simulink model "gtcs_model_and_controller"  (R2021a)
settings: Solver=VariableStepAuto  StartTime=0.0  StopTime=10  RelTol=1e-3
InitFcn:
  | load('param_motor.mat');
  | load('param_controller_2.mat');
values from neighbouring files (symbols this model uses):
  K_t = 0.0375    [param_motor.mat]
libraries: fl_lib x21, nesl_utility x13, ee_lib x10, sdl_lib x4
settings Model: Creator=ANKARA-OFIS  LastModifiedBy=ANKARA-OFIS

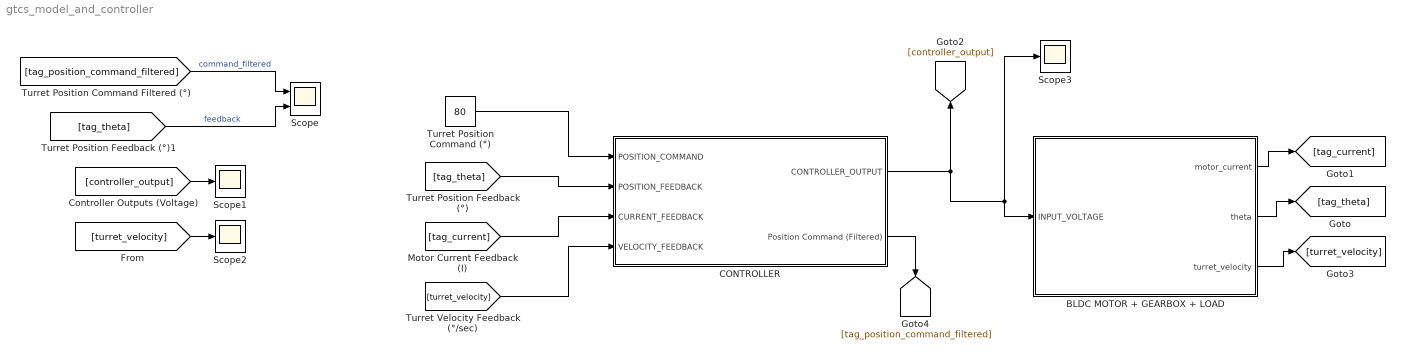
== system gtcs_model_and_controller ==
  BLDC MOTOR + GEARBOX + LOAD : Subsystem
  CONTROLLER : Subsystem
  Scope : Scope  NumInputPorts=2
  Scope1 : Scope
  Scope2 : Scope
  Scope3 : Scope
  Turret Position Command (°) : Constant  Value=80
  wires:
  Turret Position Command (°)/1 -> CONTROLLER/1(POSITION_COMMAND)
  [tag_theta] -> CONTROLLER/2(POSITION_FEEDBACK)
  [tag_current] -> CONTROLLER/3(CURRENT_FEEDBACK)
  BLDC MOTOR + GEARBOX + LOAD/2(theta) -> [tag_theta]
  BLDC MOTOR + GEARBOX + LOAD/1(motor_current) -> [tag_current]
  BLDC MOTOR + GEARBOX + LOAD/3(turret_velocity) -> [turret_velocity]
  [turret_velocity] -> CONTROLLER/4(VELOCITY_FEEDBACK)
  [turret_velocity] -> Scope2/1
  [controller_output] -> Scope1/1
  [tag_theta] -> Scope/2  "feedback"
  [tag_position_command_filtered] -> Scope/1  "command_filtered"
  CONTROLLER/2(Position Command (Filtered)) -> [tag_position_command_filtered]
  CONTROLLER/1(CONTROLLER_OUTPUT) -> Scope3/1, BLDC MOTOR + GEARBOX + LOAD/1(INPUT_VOLTAGE), [controller_output]

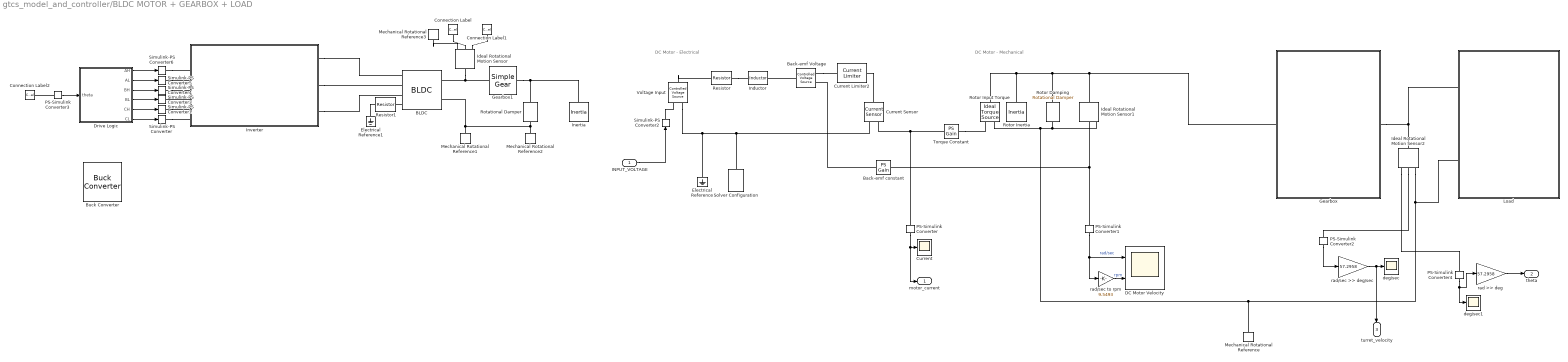
== system gtcs_model_and_controller/BLDC MOTOR + GEARBOX + LOAD ==
  note: DC Motor - Mechanical
  note: DC Motor - Electrical
  INPUT_VOLTAGE : Inport
  BLDC : ee_lib/Electromechanical/Permanent Magnet/BLDC  winding_type=ee.enum.statorconnection.wye  rotor_param=ee.enum.pmsm.backemf.trapezoidflux  pm_flux_linkage=0.03 Wb  theta_constant=pi / 12 rad  emf_max=9.6 V  DphiDtheta_tab=[0, -.1528, -.1528, .1528, .1528, 0] Wb/rad  back_emf_tab=[0, -9.6, -9.6, 9.6, 9.6, 0] V  rotor_angle_tab=[0, 7.5, 22.5, 37.5, 52.5, 60] deg  w_meas=600 rpm  nPolePairs=6  stator_param=ee.enum.statorparam.LdLqL0  machine_param=ee.enum.dqparameterization.constant  Ld=0.00022 H  Lq=0.00022 H  idVec=[-200, 0, 200] A  iqVec=[-200, 0, 200] A  LdMatrix=0.00022 * ones(3, 3) H  LqMatrix=0.00022 * ones(3, 3) H  L0=0.00016 H  Ls=0.0002 H  Lm=0 H  Ms=0.00002 H  Rs=0.013 Ohm  zero_sequence=ee.enum.park.zerosequence.include  J=0.01 kg*m^2  lam=0 N*m/(rad/s)  axes_param=ee.enum.rotorangle.daxis  i_d_specify=off  i_d_priority=None  i_d=0 A  i_d_nominal_specify=off  i_d_nominal_unit=A  i_d_nominal_value=1  i_q_specify=off  i_q_priority=None  i_q=0 A  i_q_nominal_specify=off  i_q_nominal_unit=A  i_q_nominal_value=1  torque_specify=off  torque_priority=None  torque=0 N*m  torque_nominal_specify=off  torque_nominal_unit=N*m  torque_nominal_value=1  angular_velocity_specify=off  angular_velocity_priority=High  angular_velocity=0 rpm  angular_velocity_nominal_specify=off  angular_velocity_nominal_unit=rpm  angular_velocity_nominal_value=1  angular_position_specify=off  angular_position_priority=High  angular_position=0 deg  angular_position_nominal_specify=off  angular_position_nominal_unit=deg  angular_position_nominal_value=1  loss_param=ee.enum.ironloss.none  losses_oc=[0, 0, 0] W  losses_sc=[0, 0, 0] W  f_losses=60 Hz  Isc_losses=95 A  Tmeas=298.15 K  alpha=3.93e-3 1/K  alpha_flux=-0.001 1/K  stator_thermal_mass=100 J/K  rotor_thermal_mass=200 J/K  Rm_percent_rotor=90  Rd_percent_rotor=30  temperatureA_specify=off  temperatureA_priority=High  temperatureA=25 degC  temperatureA_nominal_specify=off  temperatureA_nominal_unit=degC  temperatureA_nominal_value=1  temperatureB_specify=off  temperatureB_priority=High  temperatureB=25 degC  temperatureB_nominal_specify=off  temperatureB_nominal_unit=degC  temperatureB_nominal_value=1  temperatureC_specify=off  temperatureC_priority=High  temperatureC=25 degC  temperatureC_nominal_specify=off  temperatureC_nominal_unit=degC  temperatureC_nominal_value=1  temperatureR_specify=off  temperatureR_priority=High  temperatureR=25 degC  temperatureR_nominal_specify=off  temperatureR_nominal_unit=degC  temperatureR_nominal_value=1
      settings: SourceProductBaseCode=PS  InternalSimscapePortConfiguration="{\"Bottom\":[],\"Left\":[{\"id\":\"a\",\"label\":\"a\",\"type\":\"foundation.electrical.electrical\"},{\"id\":\"b\",\"label\":\"b\",\"type\":\"foundation.electrical.electrical\"},{\"id\":\"c\",\"label\":\"c\",\"type\":\"foundation.electrical.electrical\"},{\"id\":\"n\",\"label\":\"n\",\"type\":\"foundation.electrical.electrical\"}],\"Right\":[{\"id\":\"R\",\"label\":\"R\",\"type\":\"foundation.mechanical.rotational.rotational\"},{\"id\":\"C\",\"label\":\"C\",\"type\":\"foundation.mechanical.rotational.rotational\"}],\"Top\":[]}"
  Back-emf Voltage : fl_lib/Electrical/Electrical Sources/Controlled Voltage Source
  Back-emf constant : fl_lib/Physical Signals/Functions/PS Gain  gain=0.04 V*s/rad
  Buck Converter : ee_lib/Semiconductors & Converters/Converters/Buck Converter  device_type=ee.enum.converters.switchingdevice.ideal  Vf=0.8 V  Ron=0.001 Ohm  Rds=0.001 Ohm  Goff=1e-5 1/Ohm  Vth=6 V  Vgt=1 V  Vgt_off=-1 V  Ih=1 A  diode_param=ee.enum.converters.protectiondiode.nodynamics  diode_Vf=0.8 V  diode_Ron=0.001 Ohm  diode_Goff=1e-5 1/Ohm  diode_C=50 nF  diode_iRM=-235 A  diode_iF=300 A  diode_idot=-50 A/us  diode_trr_param=ee.enum.converters.diodetrr.trr_factor  diode_trr_factor=3  diode_trr=15 us  diode_Qrr=1500 s*uA  Lf=1e-6 H  Rl=0 Ohm  Cf=1e-7 F  Rf=1e-6 Ohm  snubber_type=ee.enum.converters.snubber.exclude  Rs=0.1 Ohm  Cs=1e-7 F  iL_specify=off  iL_priority=High  iL=0 A  iL_nominal_specify=off  iL_nominal_unit=A  iL_nominal_value=1  vc_specify=off  vc_priority=High  vc=0 V  vc_nominal_specify=off  vc_nominal_unit=V  vc_nominal_value=1
      settings: SourceProductBaseCode=PS  InternalSimscapePortConfiguration="{\"Bottom\":[],\"Left\":[{\"id\":\"G\",\"label\":\"G\",\"type\":\"input\"},{\"id\":\"p1\",\"label\":\"1+\",\"type\":\"foundation.electrical.electrical\"},{\"id\":\"n1\",\"label\":\"1-\",\"type\":\"foundation.electrical.electrical\"}],\"Right\":[{\"id\":\"p2\",\"label\":\"2+\",\"type\":\"foundation.electrical.electrical\"},{\"id\":\"n2\",\"label\":\"2-\",\"type\":\"foundation.electrical.electrical\"}],\"Top\":[]}"
  Connection Label : ConnectionLabel  Label=motor_omega
  Connection Label1 : ConnectionLabel  Label=motor_theta
  Connection Label2 : ConnectionLabel  Label=motor_theta
  Current : Scope
  Current Limiter2 : ee_lib/Semiconductors & Converters/Current Limiter  iLim=80 A  vLim=0.1 V  gLim=1e-3 1/Ohm  thermal_mass=100 J/K  initial_temperature=298.15 K
      settings: SourceProductBaseCode=PS  InternalSimscapePortConfiguration="{\"Bottom\":[],\"Left\":[{\"id\":\"p\",\"label\":\"+\",\"type\":\"foundation.electrical.electrical\"}],\"Right\":[{\"id\":\"n\",\"label\":\"-\",\"type\":\"foundation.electrical.electrical\"}],\"Top\":[]}"
  Current Sensor : fl_lib/Electrical/Electrical Sensors/Current Sensor
  DC Motor Velocity : Scope  NumInputPorts=2
  Drive Logic : MATLAB Function  TreatAsAtomicUnit=on
  Electrical Reference : fl_lib/Electrical/Electrical Elements/Electrical Reference
  Electrical Reference1 : fl_lib/Electrical/Electrical Elements/Electrical Reference
  Gearbox : Subsystem
  Gearbox1 : sdl_lib/Gears/Simple Gear  ratio=435.6  rotation_direction=sdl.enum.shaftOutputDirection.same  friction_model=sdl.enum.gear_efficiencies_load.off  mu_visc=[0, 0] N*m/(rad/s)  T_noload=0.1 N*m  T_nom=5 N*m  efficiency_nom=0.8  efficiency=0.8  temperature_TLU=[280, 300, 320] K  load_TLU=[1, 5, 10] N*m  efficiency_TLU=[.95, .9, .85]  efficiency_TLU2=[.85, .8, .75; .95, .9, .85; .85, .8, .7]  w_thr=0.01 rad/s  pwr_thr=0.001 W  thermal_mass=50 J/K  enable_faults=simscape.enum.onoff.off  efficiency_fault=0.05  external_fault=simscape.enum.onoff.off  temporal_fault=simscape.enum.onoff.off  fault_time=5 s  fault_angles=pi / 12 rad  report_fault=simscape.enum.assert.action.none  temperature_specify=off  temperature_priority=High  temperature=300 K  temperature_nominal_specify=off  temperature_nominal_unit=K  temperature_nominal_value=1
  Ideal Rotational Motion Sensor : fl_lib/Mechanical/Mechanical Sensors/Ideal Rotational Motion Sensor  wrap_angle=simscape.enum.onoff.off  offset=0 rad
  Ideal Rotational Motion Sensor1 : fl_lib/Mechanical/Mechanical Sensors/Ideal Rotational Motion Sensor  wrap_angle=simscape.enum.onoff.on  offset=0 rad
  Ideal Rotational Motion Sensor2 : fl_lib/Mechanical/Mechanical Sensors/Ideal Rotational Motion Sensor  wrap_angle=simscape.enum.onoff.off  offset=0 rad
  Inductor : ee_lib/Passive/Inductor  l=18e-6 H  L_tol=20  enable_L_tol=0  tol_distribution=1  nSigma=4  r=0 Ohm  g=1e-9 1/Ohm  enable_operating_limits=0  operating_limit_action=2  max_working_current=1 A  power_rating=1 W  enable_faults=0  fault_action=1  lambdaPercent=50  k_faulted=0.9999  turnsShort=0  openCct=0  groundShort=0  groundShortG=0 1/Ohm  tau_fault=1e-3 s  enable_temporal_fault=0  t_fault=1 s  enable_behavioral_fault=0  max_permissible_voltage=100 V  n_fail_on_voltage=1  max_permissible_current=1 A  t_fail_on_current=1 s  i_L_specify=off  i_L_priority=High  i_L=0 A  i_L_nominal_specify=off  i_L_nominal_unit=A  i_L_nominal_value=1
  Inertia : fl_lib/Mechanical/Rotational Elements/Inertia  inertia=0.01 kg*m^2  num_ports=foundation.enum.numPorts2.one  w_specify=off  w_priority=High  w=0 rad/s  w_nominal_specify=off  w_nominal_unit=rad/s  w_nominal_value=1  t_specify=off  t_priority=None  t=0 N*m  t_nominal_specify=off  t_nominal_unit=N*m  t_nominal_value=1
  Inverter : Subsystem
  Load : Subsystem
  Mechanical Rotational Reference{,1..3} (4 alike) : fl_lib/Mechanical/Rotational Elements/Mechanical Rotational Reference
  PS-Simulink Converter{,1..4} (5 alike) : nesl_utility/PS-Simulink Converter  PhysicalDomain=network_engine_domain  SubClassName=ps_output  LeftPortType=input  RightPortType=output  PseudoPeriodic=off  Frequencies=[]  Unit=inherit  AffineConversion=off
      settings: SourceProductBaseCode=PW,SS
  Resistor : fl_lib/Electrical/Electrical Elements/Resistor  R=45e-03 Ohm  i_specify=off  i_priority=None  i=0 A  i_nominal_specify=off  i_nominal_unit=A  i_nominal_value=1  v_specify=off  v_priority=None  v=0 V  v_nominal_specify=off  v_nominal_unit=V  v_nominal_value=1
  Resistor1 : fl_lib/Electrical/Electrical Elements/Resistor  R=1 Ohm  i_specify=off  i_priority=None  i=0 A  i_nominal_specify=off  i_nominal_unit=A  i_nominal_value=1  v_specify=off  v_priority=None  v=0 V  v_nominal_specify=off  v_nominal_unit=V  v_nominal_value=1
  Rotational Damper : sdl_lib/Couplings & Drives/Springs & Dampers/Rotational Damper  D=1e-3 N*m/(rad/s)  enable_faults=0  b_fault=100 N*m/(rad/s)  temporal_fault=0  fault_time=5 s  shock_fault=0  acceleration_limit=100 rad/s^2  shock_limit=1  report_fault=1
      settings: SourceProductBaseCode=LD
  Rotor Damping : fl_lib/Mechanical/Rotational Elements/Rotational Damper  D=0.0001 N*m/(rad/s)  w_specify=off  w_priority=None  w=0 rad/s  w_nominal_specify=off  w_nominal_unit=rad/s  w_nominal_value=1  t_specify=off  t_priority=None  t=0 N*m  t_nominal_specify=off  t_nominal_unit=N*m  t_nominal_value=1
  Rotor Inertia : fl_lib/Mechanical/Rotational Elements/Inertia  inertia=100 kg*mm^2  num_ports=foundation.enum.numPorts2.one  w_specify=off  w_priority=High  w=0 rad/s  w_nominal_specify=off  w_nominal_unit=rad/s  w_nominal_value=1  t_specify=off  t_priority=None  t=0 N*m  t_nominal_specify=off  t_nominal_unit=N*m  t_nominal_value=1
  Rotor Input Torque : fl_lib/Mechanical/Mechanical Sources/Ideal Torque Source
  Simulink-PS Converter{,1..6} (7 alike) : nesl_utility/Simulink-PS Converter  PhysicalDomain=network_engine_domain  SubClassName=ps_input  LeftPortType=input  RightPortType=output  PseudoPeriodic=off  Frequencies=[]  NoiseDistribution=none  NoiseParameters=[]  Unit=1  AffineConversion=off  FilteringAndDerivatives=provide  SimscapeFilterOrder=1  InputFilterTimeConstant=0.001  UdotUserProvided=0
      settings: SourceProductBaseCode=PW,SS
  Solver Configuration : nesl_utility/Solver Configuration  PhysicalDomain=network_engine_domain  SubClassName=solver  LeftPortType=input  RightPortType=generic  Tones=[]  Harmonics=[]  SimulateNoise=off  Profile=off  UseLocalSampling=off  EnableSwitchedLinearOptims=on  FrequencyDomain=off  UseCCode=off  RelTol=0.001  AbsTol=1e-06  MinStep=1e-09  ToWorkspace=off  RevertToSquareIcSolve=off  NumHomotopyIterations=100  PhasorMode=off  PhasorModeNumHarmonics=1  DoDC=off  ResidualTolerance=1e-09  UseLocalSolver=off  LocalSolverChoice=NE_BACKWARD_EULER_ADVANCER  LocalSolverSampleTime=0.001  DoFixedCost=off  MaxNonlinIter=3  MaxModeIter=2  ComputeImpulses=off  ImpulseIterations=2  LinearAlgebra=auto  EquationFormulation=NE_TIME_EF  DelaysMemoryBudget=1024  AutomaticFiltering=on  FilteringTimeConstant=0.001  PartitionStorageMethod=AS_NEEDED  PartitionMemoryBudget=1024  PartitionMethod=ROBUST
      settings: SourceProductBaseCode=PW,SS
  Torque Constant : fl_lib/Physical Signals/Functions/PS Gain  gain=K_t N*m/A
  Voltage Input : fl_lib/Electrical/Electrical Sources/Controlled Voltage Source
  deg/sec : Scope
  deg/sec1 : Scope
  rad >> deg : Gain  Gain=57.2958
  rad/sec >> deg/sec : Gain  Gain=57.2958
  rad/sec to rpm : Gain  Gain=9.5493
  motor_current : Outport
  theta : Outport  Port=2
  turret_velocity : Outport  Port=3
  wires:
  PS-Simulink Converter2/1 -> rad/sec >> deg/sec/1
  INPUT_VOLTAGE/1 -> Simulink-PS Converter2/1
  PS-Simulink Converter/1 -> motor_current/1, Current/1
  PS-Simulink Converter1/1 -> DC Motor Velocity/1, rad/sec to rpm/1  "rad/sec"
  rad/sec to rpm/1 -> DC Motor Velocity/2  "rpm"
  rad/sec >> deg/sec/1 -> turret_velocity/1, deg/sec/1
  PS-Simulink Converter4/1 -> rad >> deg/1, deg/sec1/1
  rad >> deg/1 -> theta/1
  PS-Simulink Converter3/1 -> Drive Logic/1(theta)
  Drive Logic/6(CL) -> Simulink-PS Converter/1
  Drive Logic/5(CH) -> Simulink-PS Converter1/1
  Drive Logic/4(BL) -> Simulink-PS Converter3/1
  Drive Logic/3(BH) -> Simulink-PS Converter4/1
  Drive Logic/2(AL) -> Simulink-PS Converter5/1
  Drive Logic/1(AH) -> Simulink-PS Converter6/1
  connections:
  Rotor Damping/LConn1 -- Rotor Input Torque/LConn1 -- Rotor Inertia/LConn1 -- Gearbox/LConn1 -- Ideal Rotational Motion Sensor1/LConn1
  Mechanical Rotational Reference/LConn1 -- Rotor Damping/RConn1 -- Ideal Rotational Motion Sensor1/RConn1 -- Rotor Input Torque/RConn2 -- Ideal Rotational Motion Sensor2/RConn1 -- Load/LConn2
  Ideal Rotational Motion Sensor2/RConn2 -- PS-Simulink Converter2/LConn1
  Torque Constant/RConn1 -- Rotor Input Torque/RConn1
  Ideal Rotational Motion Sensor1/RConn2 -- PS-Simulink Converter1/LConn1 -- Back-emf constant/LConn1
  Voltage Input/RConn1 -- Simulink-PS Converter2/RConn1
  Resistor/RConn1 -- Inductor/LConn1
  Current Limiter2/RConn1 -- Current Sensor/LConn1
  Voltage Input/LConn1 -- Resistor/LConn1
  Back-emf Voltage/RConn2 -- Current Limiter2/LConn1
  Torque Constant/LConn1 -- Current Sensor/RConn1 -- PS-Simulink Converter/LConn1
  Back-emf constant/RConn1 -- Back-emf Voltage/RConn1
  Back-emf Voltage/LConn1 -- Inductor/RConn1
  Electrical Reference/LConn1 -- Voltage Input/RConn2 -- Solver Configuration/RConn1 -- Current Sensor/RConn2
  Gearbox/RConn1 -- Load/LConn1 -- Ideal Rotational Motion Sensor2/LConn1
  Ideal Rotational Motion Sensor2/RConn3 -- PS-Simulink Converter4/LConn1
  Inverter/RConn2 -- BLDC/LConn2
  Inverter/RConn3 -- BLDC/LConn3
  Resistor1/LConn1 -- BLDC/LConn4
  Electrical Reference1/LConn1 -- Resistor1/RConn1
  Rotational Damper/LConn1 -- Gearbox1/RConn1 -- Inertia/LConn1
  Gearbox1/LConn1 -- Ideal Rotational Motion Sensor/LConn1 -- BLDC/RConn1
  Mechanical Rotational Reference1/LConn1 -- Rotational Damper/RConn1 -- Mechanical Rotational Reference2/LConn1 -- BLDC/RConn2
  Mechanical Rotational Reference3/LConn1 -- Ideal Rotational Motion Sensor/RConn1
  Connection Label/LConn1 -- Ideal Rotational Motion Sensor/RConn2
  Connection Label1/LConn1 -- Ideal Rotational Motion Sensor/RConn3
  Inverter/RConn1 -- BLDC/LConn1
  PS-Simulink Converter3/LConn1 -- Connection Label2/LConn1
  Simulink-PS Converter/RConn1 -- Inverter/LConn8
  Simulink-PS Converter1/RConn1 -- Inverter/LConn7
  Simulink-PS Converter3/RConn1 -- Inverter/LConn6
  Simulink-PS Converter4/RConn1 -- Inverter/LConn5
  Simulink-PS Converter5/RConn1 -- Inverter/LConn4
  Simulink-PS Converter6/RConn1 -- Inverter/LConn3

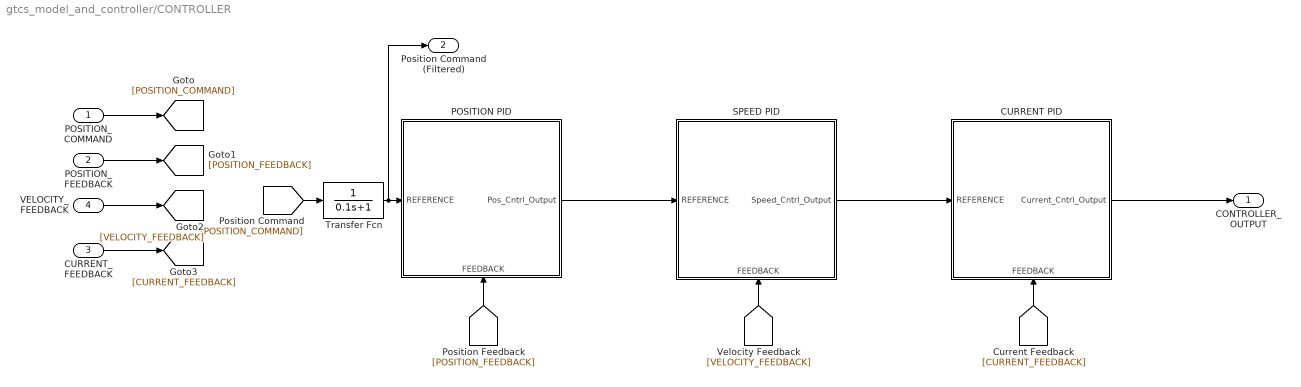
== system gtcs_model_and_controller/CONTROLLER ==
  POSITION_COMMAND : Inport
  POSITION_FEEDBACK : Inport  Port=2
  CURRENT_FEEDBACK : Inport  Port=3
  VELOCITY_FEEDBACK : Inport  Port=4
  CURRENT PID : Subsystem
      settings: PortSchema="{\"entries\":[{\"content\":{\"sides\":[{\"content\":{\"connectorIds\":[\"In1\"]},\"type\":\"ConnectorPlacement.EquallySpacedRectSide\",\"uuid\":\"40c65be9-b241-43d3-b74e-061528d6863f\"},{\"content\":{\"connectorIds\":[\"Out1\"],\"side\":\"RIGHT\"},\"type\":\"ConnectorPlacement.EquallySpacedRectSide\",\"uuid\":\"f0c37777-6186-40ca-93fa-111567e4da2a\"},{\"content\":{\"connectorIds\":[],\"side\":\"TOP\"},\"type\":\"ConnectorPlacement.EquallySpacedRectSide\",\"uuid\":\"f72b91dc-29bd-47db-bfb1-a15381258f12\"},{\"content\":{\"connectorIds\":[\"In2\"],\"side\":\"BOTTOM\"},\"type\":\"ConnectorPlacement.EquallySpacedRectSide\",\"uuid\":\"2008c998-139c-4ab5-8b80-fe5598144eb1\"}]},\"type\":\"ConnectorPlacement.EquallySpacedConnector\",\"uuid\":\"6c18c1ed-cfc3-452d-a661-af16ec8cef93\"}],\"packageUris\":[\"http://schema.mathworks.com/mf0/Connector/R2020b\"],\"version\":\"1.0\"}"
  POSITION PID : Subsystem
      settings: PortSchema="{\"entries\":[{\"content\":{\"sides\":[{\"content\":{\"connectorIds\":[\"In1\"]},\"type\":\"ConnectorPlacement.EquallySpacedRectSide\",\"uuid\":\"40c65be9-b241-43d3-b74e-061528d6863f\"},{\"content\":{\"connectorIds\":[\"Out1\"],\"side\":\"RIGHT\"},\"type\":\"ConnectorPlacement.EquallySpacedRectSide\",\"uuid\":\"f0c37777-6186-40ca-93fa-111567e4da2a\"},{\"content\":{\"connectorIds\":[],\"side\":\"TOP\"},\"type\":\"ConnectorPlacement.EquallySpacedRectSide\",\"uuid\":\"f72b91dc-29bd-47db-bfb1-a15381258f12\"},{\"content\":{\"connectorIds\":[\"In2\"],\"side\":\"BOTTOM\"},\"type\":\"ConnectorPlacement.EquallySpacedRectSide\",\"uuid\":\"2008c998-139c-4ab5-8b80-fe5598144eb1\"}]},\"type\":\"ConnectorPlacement.EquallySpacedConnector\",\"uuid\":\"6c18c1ed-cfc3-452d-a661-af16ec8cef93\"}],\"packageUris\":[\"http://schema.mathworks.com/mf0/Connector/R2020b\"],\"version\":\"1.0\"}"
  SPEED PID : Subsystem
      settings: PortSchema="{\"entries\":[{\"content\":{\"sides\":[{\"content\":{\"connectorIds\":[\"In1\"]},\"type\":\"ConnectorPlacement.EquallySpacedRectSide\",\"uuid\":\"40c65be9-b241-43d3-b74e-061528d6863f\"},{\"content\":{\"connectorIds\":[\"Out1\"],\"side\":\"RIGHT\"},\"type\":\"ConnectorPlacement.EquallySpacedRectSide\",\"uuid\":\"f0c37777-6186-40ca-93fa-111567e4da2a\"},{\"content\":{\"connectorIds\":[],\"side\":\"TOP\"},\"type\":\"ConnectorPlacement.EquallySpacedRectSide\",\"uuid\":\"f72b91dc-29bd-47db-bfb1-a15381258f12\"},{\"content\":{\"connectorIds\":[\"In2\"],\"side\":\"BOTTOM\"},\"type\":\"ConnectorPlacement.EquallySpacedRectSide\",\"uuid\":\"2008c998-139c-4ab5-8b80-fe5598144eb1\"}]},\"type\":\"ConnectorPlacement.EquallySpacedConnector\",\"uuid\":\"6c18c1ed-cfc3-452d-a661-af16ec8cef93\"}],\"packageUris\":[\"http://schema.mathworks.com/mf0/Connector/R2020b\"],\"version\":\"1.0\"}"
  Transfer Fcn : TransferFcn  Denominator=[0.1 1]
  CONTROLLER_OUTPUT : Outport
  Position Command (Filtered) : Outport  Port=2
  wires:
  POSITION_COMMAND/1 -> [POSITION_COMMAND]
  POSITION_FEEDBACK/1 -> [POSITION_FEEDBACK]
  VELOCITY_FEEDBACK/1 -> [VELOCITY_FEEDBACK]
  CURRENT_FEEDBACK/1 -> [CURRENT_FEEDBACK]
  [POSITION_COMMAND] -> Transfer Fcn/1
  [POSITION_FEEDBACK] -> POSITION PID/2(FEEDBACK)
  [VELOCITY_FEEDBACK] -> SPEED PID/2(FEEDBACK)
  [CURRENT_FEEDBACK] -> CURRENT PID/2(FEEDBACK)
  POSITION PID/1(Pos_Cntrl_Output) -> SPEED PID/1(REFERENCE)
  CURRENT PID/1(Current_Cntrl_Output) -> CONTROLLER_OUTPUT/1
  SPEED PID/1(Speed_Cntrl_Output) -> CURRENT PID/1(REFERENCE)
  Transfer Fcn/1 -> Position Command (Filtered)/1, POSITION PID/1(REFERENCE)

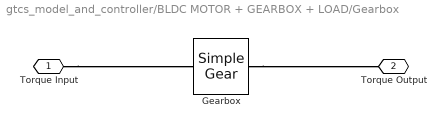
== system gtcs_model_and_controller/BLDC MOTOR + GEARBOX + LOAD/Gearbox ==
  Gearbox : sdl_lib/Gears/Simple Gear  ratio=435.6  rotation_direction=sdl.enum.shaftOutputDirection.same  friction_model=sdl.enum.gear_efficiencies_load.off  mu_visc=[0, 0] N*m/(rad/s)  T_noload=0.1 N*m  T_nom=5 N*m  efficiency_nom=0.8  efficiency=0.8  temperature_TLU=[280, 300, 320] K  load_TLU=[1, 5, 10] N*m  efficiency_TLU=[.95, .9, .85]  efficiency_TLU2=[.85, .8, .75; .95, .9, .85; .85, .8, .7]  w_thr=0.01 rad/s  pwr_thr=0.001 W  thermal_mass=50 J/K  enable_faults=simscape.enum.onoff.off  efficiency_fault=0.05  external_fault=simscape.enum.onoff.off  temporal_fault=simscape.enum.onoff.off  fault_time=5 s  fault_angles=pi / 12 rad  report_fault=simscape.enum.assert.action.none  temperature_specify=off  temperature_priority=High  temperature=300 K  temperature_nominal_specify=off  temperature_nominal_unit=K  temperature_nominal_value=1
  Torque Input : PMIOPort  Side=Left
  Torque Output : PMIOPort  Port=2  Side=Right
  connections:
  Gearbox/RConn1 -- Torque Output/RConn1
  Torque Input/RConn1 -- Gearbox/LConn1

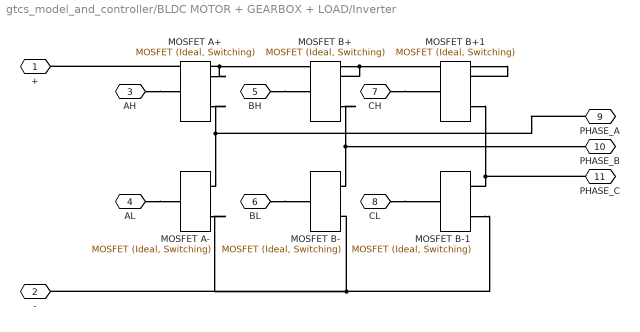
== system gtcs_model_and_controller/BLDC MOTOR + GEARBOX + LOAD/Inverter ==
  MOSFET A+ : ee_lib/Semiconductors & Converters/MOSFET (Ideal, Switching)  Rds=0.01 Ohm  Goff=1e-6 1/Ohm  Vth=2 V  diode_param=ee.enum.converters.protectiondiode.none  diode_Vf=0.8 V  diode_Ron=0.001 Ohm  diode_Goff=1e-5 1/Ohm  diode_C=50e-9 F  diode_iRM=-235 A  diode_iF=300 A  diode_idot=-50 A/us  diode_trr_param=ee.enum.converters.diodetrr.trr_factor  diode_trr_factor=3  diode_trr=15 us  diode_Qrr=1500 s*uA  thermal_loss_option=ee.enum.converters.thermalLossOption.constantvalues  Von_data=[0, 1.1, 1.3, 1.45, 1.75, 2.25, 2.7; 0, 1, 1.15, 1.35, 1.7, 2.35, 3] V  Eon_data=[0, .29, 1.43, 2.86, 5.71, 13.14, 22.86; 0, .57, 2.63, 5.14, 10.29, 20.57, 30.29] * 1e-3 J  Eoff_data=[0, .21, 1.07, 2.14, 4.29, 9.86, 17.14; 0, .43, 1.97, 3.86, 7.71, 15.43, 22.71] * 1e-3 J  Tj=[298.15, 398.15] K  Iout_data=[0, 10, 50, 100, 200, 400, 600] A  Eon_scalar=22.86e-3 J  Eoff_scalar=17.14e-3 J  Voff=300 V  Iout_scalar=600 A  diodeModelType=ee.enum.converters.diodeModelType.pwl  diode_IfMat=[.07, .12, .19, 1.75, 4.24, 7.32, 11.2; .16, .3, .72, 2.14, 4.02, 6.35, 9.12] A  diode_TjVec=[25, 125] degC  diode_VfVec=[.5, .7, .9, 1.3, 1.7, 2.1, 2.5] V  thermal_network_parameterization=ee.enum.thermalNetworkTopology.external  Rth=[.03, .2] K/W  Rth_Foster=[.03, .2] K/W  thermal_mass_parameterization=ee.enum.thermalNetwork.timeconstant  thermal_mass=[3, 25] J/K  thermal_mass_Foster=[33, 50] J/K  thermal_time_constant=[.1, 5] s  thermal_time_constant_Foster=[1, 10] s  thermal_mass_initial_temperatures=[25, 25] degC  junction_thermal_mass=0.1 J/K  vT_specify=off  vT_priority=None  vT=0 V  vT_nominal_specify=off  vT_nominal_unit=V  vT_nominal_value=1  Qj_specify=off  Qj_priority=None  Qj=0 W  Qj_nominal_specify=off  Qj_nominal_unit=W  Qj_nominal_value=1  junction_temperature_specify=off  junction_temperature_priority=None  junction_temperature=25 degC  junction_temperature_nominal_specify=off  junction_temperature_nominal_unit=degC  junction_temperature_nominal_value=1
  MOSFET A- : ee_lib/Semiconductors & Converters/MOSFET (Ideal, Switching)  Rds=0.01 Ohm  Goff=1e-6 1/Ohm  Vth=2 V  diode_param=ee.enum.converters.protectiondiode.none  diode_Vf=0.8 V  diode_Ron=0.001 Ohm  diode_Goff=1e-5 1/Ohm  diode_C=50e-9 F  diode_iRM=-235 A  diode_iF=300 A  diode_idot=-50 A/us  diode_trr_param=ee.enum.converters.diodetrr.trr_factor  diode_trr_factor=3  diode_trr=15 us  diode_Qrr=1500 s*uA  thermal_loss_option=ee.enum.converters.thermalLossOption.constantvalues  Von_data=[0, 1.1, 1.3, 1.45, 1.75, 2.25, 2.7; 0, 1, 1.15, 1.35, 1.7, 2.35, 3] V  Eon_data=[0, .29, 1.43, 2.86, 5.71, 13.14, 22.86; 0, .57, 2.63, 5.14, 10.29, 20.57, 30.29] * 1e-3 J  Eoff_data=[0, .21, 1.07, 2.14, 4.29, 9.86, 17.14; 0, .43, 1.97, 3.86, 7.71, 15.43, 22.71] * 1e-3 J  Tj=[298.15, 398.15] K  Iout_data=[0, 10, 50, 100, 200, 400, 600] A  Eon_scalar=22.86e-3 J  Eoff_scalar=17.14e-3 J  Voff=300 V  Iout_scalar=600 A  diodeModelType=ee.enum.converters.diodeModelType.pwl  diode_IfMat=[.07, .12, .19, 1.75, 4.24, 7.32, 11.2; .16, .3, .72, 2.14, 4.02, 6.35, 9.12] A  diode_TjVec=[25, 125] degC  diode_VfVec=[.5, .7, .9, 1.3, 1.7, 2.1, 2.5] V  thermal_network_parameterization=ee.enum.thermalNetworkTopology.external  Rth=[.03, .2] K/W  Rth_Foster=[.03, .2] K/W  thermal_mass_parameterization=ee.enum.thermalNetwork.timeconstant  thermal_mass=[3, 25] J/K  thermal_mass_Foster=[33, 50] J/K  thermal_time_constant=[.1, 5] s  thermal_time_constant_Foster=[1, 10] s  thermal_mass_initial_temperatures=[25, 25] degC  junction_thermal_mass=0.1 J/K  vT_specify=off  vT_priority=None  vT=0 V  vT_nominal_specify=off  vT_nominal_unit=V  vT_nominal_value=1  Qj_specify=off  Qj_priority=None  Qj=0 W  Qj_nominal_specify=off  Qj_nominal_unit=W  Qj_nominal_value=1  junction_temperature_specify=off  junction_temperature_priority=None  junction_temperature=25 degC  junction_temperature_nominal_specify=off  junction_temperature_nominal_unit=degC  junction_temperature_nominal_value=1
  MOSFET B+ : ee_lib/Semiconductors & Converters/MOSFET (Ideal, Switching)  Rds=0.01 Ohm  Goff=1e-6 1/Ohm  Vth=2 V  diode_param=ee.enum.converters.protectiondiode.none  diode_Vf=0.8 V  diode_Ron=0.001 Ohm  diode_Goff=1e-5 1/Ohm  diode_C=50e-9 F  diode_iRM=-235 A  diode_iF=300 A  diode_idot=-50 A/us  diode_trr_param=ee.enum.converters.diodetrr.trr_factor  diode_trr_factor=3  diode_trr=15 us  diode_Qrr=1500 s*uA  thermal_loss_option=ee.enum.converters.thermalLossOption.constantvalues  Von_data=[0, 1.1, 1.3, 1.45, 1.75, 2.25, 2.7; 0, 1, 1.15, 1.35, 1.7, 2.35, 3] V  Eon_data=[0, .29, 1.43, 2.86, 5.71, 13.14, 22.86; 0, .57, 2.63, 5.14, 10.29, 20.57, 30.29] * 1e-3 J  Eoff_data=[0, .21, 1.07, 2.14, 4.29, 9.86, 17.14; 0, .43, 1.97, 3.86, 7.71, 15.43, 22.71] * 1e-3 J  Tj=[298.15, 398.15] K  Iout_data=[0, 10, 50, 100, 200, 400, 600] A  Eon_scalar=22.86e-3 J  Eoff_scalar=17.14e-3 J  Voff=300 V  Iout_scalar=600 A  diodeModelType=ee.enum.converters.diodeModelType.pwl  diode_IfMat=[.07, .12, .19, 1.75, 4.24, 7.32, 11.2; .16, .3, .72, 2.14, 4.02, 6.35, 9.12] A  diode_TjVec=[25, 125] degC  diode_VfVec=[.5, .7, .9, 1.3, 1.7, 2.1, 2.5] V  thermal_network_parameterization=ee.enum.thermalNetworkTopology.external  Rth=[.03, .2] K/W  Rth_Foster=[.03, .2] K/W  thermal_mass_parameterization=ee.enum.thermalNetwork.timeconstant  thermal_mass=[3, 25] J/K  thermal_mass_Foster=[33, 50] J/K  thermal_time_constant=[.1, 5] s  thermal_time_constant_Foster=[1, 10] s  thermal_mass_initial_temperatures=[25, 25] degC  junction_thermal_mass=0.1 J/K  vT_specify=off  vT_priority=None  vT=0 V  vT_nominal_specify=off  vT_nominal_unit=V  vT_nominal_value=1  Qj_specify=off  Qj_priority=None  Qj=0 W  Qj_nominal_specify=off  Qj_nominal_unit=W  Qj_nominal_value=1  junction_temperature_specify=off  junction_temperature_priority=None  junction_temperature=25 degC  junction_temperature_nominal_specify=off  junction_temperature_nominal_unit=degC  junction_temperature_nominal_value=1
  MOSFET B+1 : ee_lib/Semiconductors & Converters/MOSFET (Ideal, Switching)  Rds=0.01 Ohm  Goff=1e-6 1/Ohm  Vth=2 V  diode_param=ee.enum.converters.protectiondiode.none  diode_Vf=0.8 V  diode_Ron=0.001 Ohm  diode_Goff=1e-5 1/Ohm  diode_C=50e-9 F  diode_iRM=-235 A  diode_iF=300 A  diode_idot=-50 A/us  diode_trr_param=ee.enum.converters.diodetrr.trr_factor  diode_trr_factor=3  diode_trr=15 us  diode_Qrr=1500 s*uA  thermal_loss_option=ee.enum.converters.thermalLossOption.constantvalues  Von_data=[0, 1.1, 1.3, 1.45, 1.75, 2.25, 2.7; 0, 1, 1.15, 1.35, 1.7, 2.35, 3] V  Eon_data=[0, .29, 1.43, 2.86, 5.71, 13.14, 22.86; 0, .57, 2.63, 5.14, 10.29, 20.57, 30.29] * 1e-3 J  Eoff_data=[0, .21, 1.07, 2.14, 4.29, 9.86, 17.14; 0, .43, 1.97, 3.86, 7.71, 15.43, 22.71] * 1e-3 J  Tj=[298.15, 398.15] K  Iout_data=[0, 10, 50, 100, 200, 400, 600] A  Eon_scalar=22.86e-3 J  Eoff_scalar=17.14e-3 J  Voff=300 V  Iout_scalar=600 A  diodeModelType=ee.enum.converters.diodeModelType.pwl  diode_IfMat=[.07, .12, .19, 1.75, 4.24, 7.32, 11.2; .16, .3, .72, 2.14, 4.02, 6.35, 9.12] A  diode_TjVec=[25, 125] degC  diode_VfVec=[.5, .7, .9, 1.3, 1.7, 2.1, 2.5] V  thermal_network_parameterization=ee.enum.thermalNetworkTopology.external  Rth=[.03, .2] K/W  Rth_Foster=[.03, .2] K/W  thermal_mass_parameterization=ee.enum.thermalNetwork.timeconstant  thermal_mass=[3, 25] J/K  thermal_mass_Foster=[33, 50] J/K  thermal_time_constant=[.1, 5] s  thermal_time_constant_Foster=[1, 10] s  thermal_mass_initial_temperatures=[25, 25] degC  junction_thermal_mass=0.1 J/K  vT_specify=off  vT_priority=None  vT=0 V  vT_nominal_specify=off  vT_nominal_unit=V  vT_nominal_value=1  Qj_specify=off  Qj_priority=None  Qj=0 W  Qj_nominal_specify=off  Qj_nominal_unit=W  Qj_nominal_value=1  junction_temperature_specify=off  junction_temperature_priority=None  junction_temperature=25 degC  junction_temperature_nominal_specify=off  junction_temperature_nominal_unit=degC  junction_temperature_nominal_value=1
  MOSFET B- : ee_lib/Semiconductors & Converters/MOSFET (Ideal, Switching)  Rds=0.01 Ohm  Goff=1e-6 1/Ohm  Vth=2 V  diode_param=ee.enum.converters.protectiondiode.none  diode_Vf=0.8 V  diode_Ron=0.001 Ohm  diode_Goff=1e-5 1/Ohm  diode_C=50e-9 F  diode_iRM=-235 A  diode_iF=300 A  diode_idot=-50 A/us  diode_trr_param=ee.enum.converters.diodetrr.trr_factor  diode_trr_factor=3  diode_trr=15 us  diode_Qrr=1500 s*uA  thermal_loss_option=ee.enum.converters.thermalLossOption.constantvalues  Von_data=[0, 1.1, 1.3, 1.45, 1.75, 2.25, 2.7; 0, 1, 1.15, 1.35, 1.7, 2.35, 3] V  Eon_data=[0, .29, 1.43, 2.86, 5.71, 13.14, 22.86; 0, .57, 2.63, 5.14, 10.29, 20.57, 30.29] * 1e-3 J  Eoff_data=[0, .21, 1.07, 2.14, 4.29, 9.86, 17.14; 0, .43, 1.97, 3.86, 7.71, 15.43, 22.71] * 1e-3 J  Tj=[298.15, 398.15] K  Iout_data=[0, 10, 50, 100, 200, 400, 600] A  Eon_scalar=22.86e-3 J  Eoff_scalar=17.14e-3 J  Voff=300 V  Iout_scalar=600 A  diodeModelType=ee.enum.converters.diodeModelType.pwl  diode_IfMat=[.07, .12, .19, 1.75, 4.24, 7.32, 11.2; .16, .3, .72, 2.14, 4.02, 6.35, 9.12] A  diode_TjVec=[25, 125] degC  diode_VfVec=[.5, .7, .9, 1.3, 1.7, 2.1, 2.5] V  thermal_network_parameterization=ee.enum.thermalNetworkTopology.external  Rth=[.03, .2] K/W  Rth_Foster=[.03, .2] K/W  thermal_mass_parameterization=ee.enum.thermalNetwork.timeconstant  thermal_mass=[3, 25] J/K  thermal_mass_Foster=[33, 50] J/K  thermal_time_constant=[.1, 5] s  thermal_time_constant_Foster=[1, 10] s  thermal_mass_initial_temperatures=[25, 25] degC  junction_thermal_mass=0.1 J/K  vT_specify=off  vT_priority=None  vT=0 V  vT_nominal_specify=off  vT_nominal_unit=V  vT_nominal_value=1  Qj_specify=off  Qj_priority=None  Qj=0 W  Qj_nominal_specify=off  Qj_nominal_unit=W  Qj_nominal_value=1  junction_temperature_specify=off  junction_temperature_priority=None  junction_temperature=25 degC  junction_temperature_nominal_specify=off  junction_temperature_nominal_unit=degC  junction_temperature_nominal_value=1
  MOSFET B-1 : ee_lib/Semiconductors & Converters/MOSFET (Ideal, Switching)  Rds=0.01 Ohm  Goff=1e-6 1/Ohm  Vth=2 V  diode_param=ee.enum.converters.protectiondiode.none  diode_Vf=0.8 V  diode_Ron=0.001 Ohm  diode_Goff=1e-5 1/Ohm  diode_C=50e-9 F  diode_iRM=-235 A  diode_iF=300 A  diode_idot=-50 A/us  diode_trr_param=ee.enum.converters.diodetrr.trr_factor  diode_trr_factor=3  diode_trr=15 us  diode_Qrr=1500 s*uA  thermal_loss_option=ee.enum.converters.thermalLossOption.constantvalues  Von_data=[0, 1.1, 1.3, 1.45, 1.75, 2.25, 2.7; 0, 1, 1.15, 1.35, 1.7, 2.35, 3] V  Eon_data=[0, .29, 1.43, 2.86, 5.71, 13.14, 22.86; 0, .57, 2.63, 5.14, 10.29, 20.57, 30.29] * 1e-3 J  Eoff_data=[0, .21, 1.07, 2.14, 4.29, 9.86, 17.14; 0, .43, 1.97, 3.86, 7.71, 15.43, 22.71] * 1e-3 J  Tj=[298.15, 398.15] K  Iout_data=[0, 10, 50, 100, 200, 400, 600] A  Eon_scalar=22.86e-3 J  Eoff_scalar=17.14e-3 J  Voff=300 V  Iout_scalar=600 A  diodeModelType=ee.enum.converters.diodeModelType.pwl  diode_IfMat=[.07, .12, .19, 1.75, 4.24, 7.32, 11.2; .16, .3, .72, 2.14, 4.02, 6.35, 9.12] A  diode_TjVec=[25, 125] degC  diode_VfVec=[.5, .7, .9, 1.3, 1.7, 2.1, 2.5] V  thermal_network_parameterization=ee.enum.thermalNetworkTopology.external  Rth=[.03, .2] K/W  Rth_Foster=[.03, .2] K/W  thermal_mass_parameterization=ee.enum.thermalNetwork.timeconstant  thermal_mass=[3, 25] J/K  thermal_mass_Foster=[33, 50] J/K  thermal_time_constant=[.1, 5] s  thermal_time_constant_Foster=[1, 10] s  thermal_mass_initial_temperatures=[25, 25] degC  junction_thermal_mass=0.1 J/K  vT_specify=off  vT_priority=None  vT=0 V  vT_nominal_specify=off  vT_nominal_unit=V  vT_nominal_value=1  Qj_specify=off  Qj_priority=None  Qj=0 W  Qj_nominal_specify=off  Qj_nominal_unit=W  Qj_nominal_value=1  junction_temperature_specify=off  junction_temperature_priority=None  junction_temperature=25 degC  junction_temperature_nominal_specify=off  junction_temperature_nominal_unit=degC  junction_temperature_nominal_value=1
  + : PMIOPort  Side=Left
  - : PMIOPort  Port=2  Side=Left
  AH : PMIOPort  Port=3  Side=Left
  AL : PMIOPort  Port=4  Side=Left
  BH : PMIOPort  Port=5  Side=Left
  BL : PMIOPort  Port=6  Side=Left
  CH : PMIOPort  Port=7  Side=Left
  CL : PMIOPort  Port=8  Side=Left
  PHASE_A : PMIOPort  Port=9  Side=Right
  PHASE_B : PMIOPort  Port=10  Side=Right
  PHASE_C : PMIOPort  Port=11  Side=Right
  connections:
  AL/RConn1 -- MOSFET A-/LConn1
  MOSFET A+/RConn1 -- MOSFET B+/RConn1 -- MOSFET B+1/RConn1 -- +/RConn1
  MOSFET B+/RConn2 -- PHASE_B/RConn1 -- MOSFET B-/RConn1
  MOSFET B-1/RConn2 -- -/RConn1 -- MOSFET A-/RConn2 -- MOSFET B-/RConn2
  BH/RConn1 -- MOSFET B+/LConn1
  MOSFET B+1/RConn2 -- PHASE_C/RConn1 -- MOSFET B-1/RConn1
  MOSFET A+/RConn2 -- PHASE_A/RConn1 -- MOSFET A-/RConn1
  CL/RConn1 -- MOSFET B-1/LConn1
  CH/RConn1 -- MOSFET B+1/LConn1
  AH/RConn1 -- MOSFET A+/LConn1
  BL/RConn1 -- MOSFET B-/LConn1

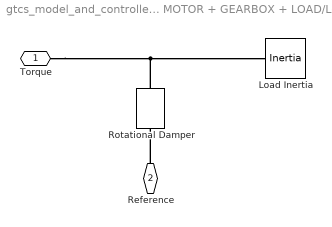
== system gtcs_model_and_controller/BLDC MOTOR + GEARBOX + LOAD/Load ==
  Load Inertia : fl_lib/Mechanical/Rotational Elements/Inertia  inertia=257 kg*m^2  num_ports=foundation.enum.numPorts2.one  w_specify=off  w_priority=High  w=0 rad/s  w_nominal_specify=off  w_nominal_unit=rad/s  w_nominal_value=1  t_specify=off  t_priority=None  t=0 N*m  t_nominal_specify=off  t_nominal_unit=N*m  t_nominal_value=1
  Rotational Damper : sdl_lib/Couplings & Drives/Springs & Dampers/Rotational Damper  D=0.1 N*m/(rad/s)  enable_faults=0  b_fault=100 N*m/(rad/s)  temporal_fault=0  fault_time=5 s  shock_fault=0  acceleration_limit=100 rad/s^2  shock_limit=1  report_fault=1
      settings: SourceProductBaseCode=LD
  Torque : PMIOPort  Side=Left
  Reference : PMIOPort  Port=2  Side=Left
  connections:
  Torque/RConn1 -- Rotational Damper/LConn1 -- Load Inertia/LConn1
  Reference/RConn1 -- Rotational Damper/RConn1

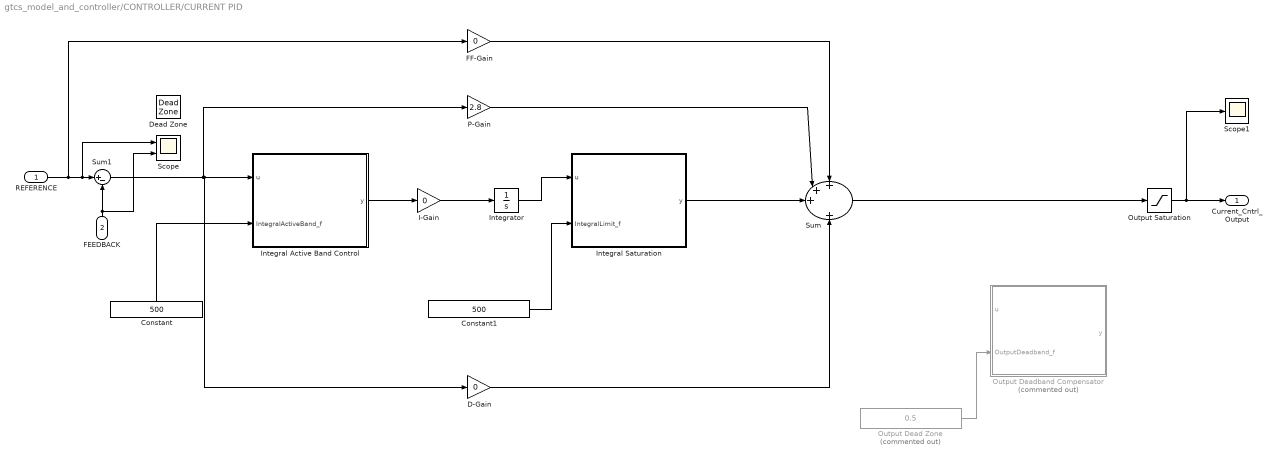
== system gtcs_model_and_controller/CONTROLLER/CURRENT PID ==
  REFERENCE : Inport
  FEEDBACK : Inport  Port=2
  Constant : Constant  Value=500
  Constant1 : Constant  Value=500
  D-Gain : Gain  Gain=0
  Dead Zone : DeadZone  SaturateOnIntegerOverflow=on
  FF-Gain : Gain  Gain=0
  I-Gain : Gain  Gain=0
  Integral Active Band Control : MATLAB Function  TreatAsAtomicUnit=on
  Integral Saturation : MATLAB Function  TreatAsAtomicUnit=on
  Integrator : Integrator
  Output Dead Zone : Constant  Commented=on  Value=0.5
  Output Deadband Compensator : MATLAB Function  Commented=on  TreatAsAtomicUnit=on
  Output Saturation : Saturate  UpperLimit=28  LowerLimit=-28
  P-Gain : Gain  Gain=2.8
  Scope : Scope  NumInputPorts=2
  Scope1 : Scope
  Sum : Sum  Inputs=+++|+
  Sum1 : Sum  Inputs=|+-
  Current_Cntrl_Output : Outport
  wires:
  Output Saturation/1 -> Scope1/1, Current_Cntrl_Output/1
  FEEDBACK/1 -> Scope/2, Sum1/2
  REFERENCE/1 -> FF-Gain/1, Scope/1, Sum1/1
  Sum1/1 -> D-Gain/1, Integral Active Band Control/1(u), P-Gain/1
  Constant/1 -> Integral Active Band Control/2(IntegralActiveBand_f)
  I-Gain/1 -> Integrator/1
  Integral Active Band Control/1(y) -> I-Gain/1
  Integrator/1 -> Integral Saturation/1(u)
  Constant1/1 -> Integral Saturation/2(IntegralLimit_f)
  Integral Saturation/1(y) -> Sum/3
  P-Gain/1 -> Sum/2
  FF-Gain/1 -> Sum/1
  D-Gain/1 -> Sum/4
  Sum/1 -> Output Saturation/1
  Output Dead Zone/1 -> Output Deadband Compensator/2(OutputDeadband_f)

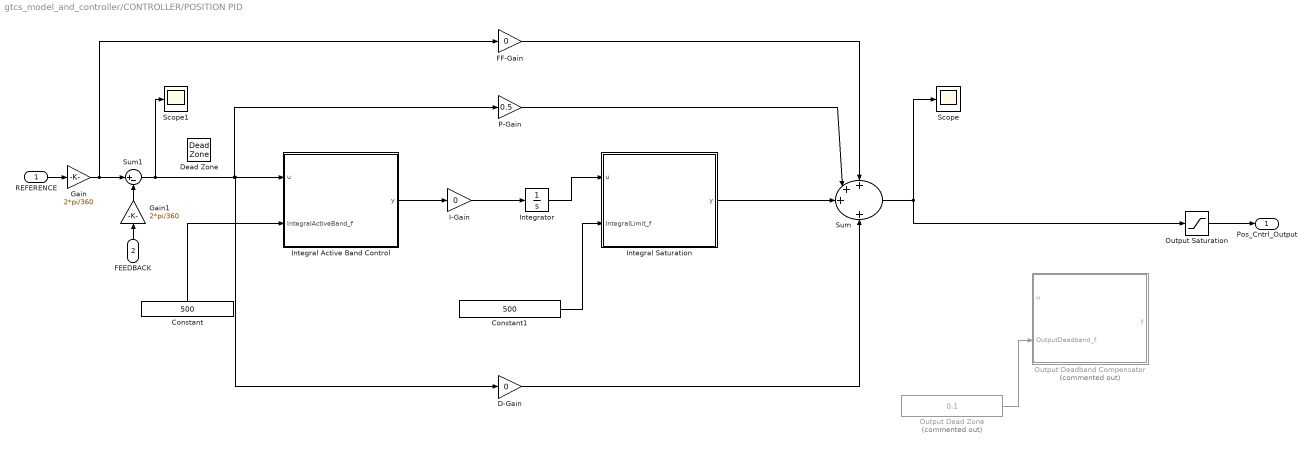
== system gtcs_model_and_controller/CONTROLLER/POSITION PID ==
  REFERENCE : Inport
  FEEDBACK : Inport  Port=2
  Constant : Constant  Value=500
  Constant1 : Constant  Value=500
  D-Gain : Gain  Gain=0
  Dead Zone : DeadZone  LowerValue=-0.01  UpperValue=0.01  SaturateOnIntegerOverflow=on
  FF-Gain : Gain  Gain=0
  Gain : Gain  Gain=2*pi/360
  Gain1 : Gain  Gain=2*pi/360
  I-Gain : Gain  Gain=0
  Integral Active Band Control : MATLAB Function  TreatAsAtomicUnit=on
  Integral Saturation : MATLAB Function  TreatAsAtomicUnit=on
  Integrator : Integrator
  Output Dead Zone : Constant  Commented=on  Value=0.1
  Output Deadband Compensator : MATLAB Function  Commented=on  TreatAsAtomicUnit=on
  Output Saturation : Saturate  UpperLimit=1.57  LowerLimit=-1.57
  P-Gain : Gain  Gain=0.5
  Scope : Scope
  Scope1 : Scope
  Sum : Sum  Inputs=+++|+
  Sum1 : Sum  Inputs=|+-
  Pos_Cntrl_Output : Outport
  wires:
  Output Saturation/1 -> Pos_Cntrl_Output/1
  FEEDBACK/1 -> Gain1/1
  REFERENCE/1 -> Gain/1
  Sum1/1 -> Scope1/1, D-Gain/1, Integral Active Band Control/1(u), P-Gain/1
  Constant/1 -> Integral Active Band Control/2(IntegralActiveBand_f)
  I-Gain/1 -> Integrator/1
  Integral Active Band Control/1(y) -> I-Gain/1
  Integrator/1 -> Integral Saturation/1(u)
  Constant1/1 -> Integral Saturation/2(IntegralLimit_f)
  Integral Saturation/1(y) -> Sum/3
  P-Gain/1 -> Sum/2
  FF-Gain/1 -> Sum/1
  D-Gain/1 -> Sum/4
  Sum/1 -> Output Saturation/1, Scope/1
  Gain/1 -> FF-Gain/1, Sum1/1
  Gain1/1 -> Sum1/2
  Output Dead Zone/1 -> Output Deadband Compensator/2(OutputDeadband_f)

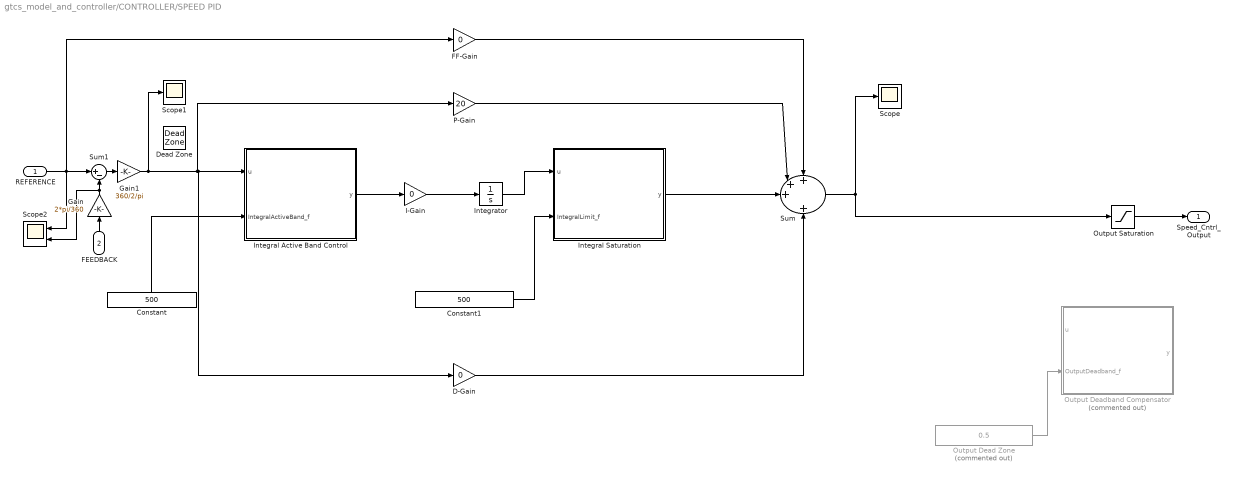
== system gtcs_model_and_controller/CONTROLLER/SPEED PID ==
  REFERENCE : Inport
  FEEDBACK : Inport  Port=2
  Constant : Constant  Value=500
  Constant1 : Constant  Value=500
  D-Gain : Gain  Gain=0
  Dead Zone : DeadZone  LowerValue=-0.1  UpperValue=0.1  SaturateOnIntegerOverflow=on
  FF-Gain : Gain  Gain=0
  Gain : Gain  Gain=2*pi/360
  Gain1 : Gain  Gain=360/2/pi
  I-Gain : Gain  Gain=0
  Integral Active Band Control : MATLAB Function  TreatAsAtomicUnit=on
  Integral Saturation : MATLAB Function  TreatAsAtomicUnit=on
  Integrator : Integrator
  Output Dead Zone : Constant  Commented=on  Value=0.5
  Output Deadband Compensator : MATLAB Function  Commented=on  TreatAsAtomicUnit=on
  Output Saturation : Saturate  UpperLimit=80  LowerLimit=-80
  P-Gain : Gain  Gain=20
  Scope : Scope
  Scope1 : Scope
  Scope2 : Scope  NumInputPorts=2
  Sum : Sum  Inputs=+++|+
  Sum1 : Sum  Inputs=|+-
  Speed_Cntrl_Output : Outport
  wires:
  Output Saturation/1 -> Speed_Cntrl_Output/1
  FEEDBACK/1 -> Gain/1
  REFERENCE/1 -> Scope2/1, FF-Gain/1, Sum1/1
  Sum1/1 -> Gain1/1
  Constant/1 -> Integral Active Band Control/2(IntegralActiveBand_f)
  I-Gain/1 -> Integrator/1
  Integral Active Band Control/1(y) -> I-Gain/1
  Integrator/1 -> Integral Saturation/1(u)
  Constant1/1 -> Integral Saturation/2(IntegralLimit_f)
  Integral Saturation/1(y) -> Sum/3
  P-Gain/1 -> Sum/2
  FF-Gain/1 -> Sum/1
  D-Gain/1 -> Sum/4
  Sum/1 -> Output Saturation/1, Scope/1
  Output Dead Zone/1 -> Output Deadband Compensator/2(OutputDeadband_f)
  Gain/1 -> Scope2/2, Sum1/2
  Gain1/1 -> Scope1/1, D-Gain/1, Integral Active Band Control/1(u), P-Gain/1

== matlab function gtcs_model_and_controller/CONTROLLER/SPEED PID/Integral Active Band Control ==
  data: u input; y output; IntegralActiveBand_f input
function y = IntegralActiveBandControl(u, IntegralActiveBand_f)
    if abs(u) <= IntegralActiveBand_f
        y = u;
    else
        y = 0;
    end
end

== matlab function gtcs_model_and_controller/CONTROLLER/SPEED PID/Integral Saturation ==
  data: u input; y output; IntegralLimit_f input
function y = IntegralSaturation(u, IntegralLimit_f)
    if u==0
        multiplier = 1;
    else
        multiplier = floor(u/abs(u));
    end
    if abs(u) < IntegralLimit_f
        y = u;
    else
        y = IntegralLimit_f * multiplier;
    end
end

== matlab function gtcs_model_and_controller/CONTROLLER/SPEED PID/Output Deadband Compensator ==
  data: u input; y output; OutputDeadband_f input
function y = Output_Deadband_Compensator(u, OutputDeadband_f)
    if u==0
        multiplier = 1;
    else
        multiplier = floor(u/abs(u));
    end
    if abs(u) == 0
        y = 0;
    else
        y = u + OutputDeadband_f * multiplier;
    end
end

== matlab function gtcs_model_and_controller/CONTROLLER/POSITION PID/Integral Active Band Control ==
  data: u input; y output; IntegralActiveBand_f input
function y = IntegralActiveBandControl(u, IntegralActiveBand_f)
    if abs(u) <= IntegralActiveBand_f
        y = u;
    else
        y = 0;
    end
end

== matlab function gtcs_model_and_controller/CONTROLLER/POSITION PID/Integral Saturation ==
  data: u input; y output; IntegralLimit_f input
function y = IntegralSaturation(u, IntegralLimit_f)
    if u==0
        multiplier = 1;
    else
        multiplier = floor(u/abs(u));
    end
    if abs(u) < IntegralLimit_f
        y = u;
    else
        y = IntegralLimit_f * multiplier;
    end
end

== matlab function gtcs_model_and_controller/CONTROLLER/POSITION PID/Output Deadband Compensator ==
  data: u input; y output; OutputDeadband_f input
function y = Output_Deadband_Compensator(u, OutputDeadband_f)
    if u==0
        multiplier = 1;
    else
        multiplier = floor(u/abs(u));
    end
    if abs(u) == 0
        y = 0;
    else
        y = u + OutputDeadband_f * multiplier;
    end
end

== matlab function gtcs_model_and_controller/CONTROLLER/CURRENT PID/Integral Active Band Control ==
  data: u input; y output; IntegralActiveBand_f input
function y = IntegralActiveBandControl(u, IntegralActiveBand_f)
    if abs(u) <= IntegralActiveBand_f
        y = u;
    else
        y = 0;
    end
end

== matlab function gtcs_model_and_controller/CONTROLLER/CURRENT PID/Integral Saturation ==
  data: u input; y output; IntegralLimit_f input
function y = IntegralSaturation(u, IntegralLimit_f)
    if u==0
        multiplier = 1;
    else
        multiplier = floor(u/abs(u));
    end
    if abs(u) < IntegralLimit_f
        y = u;
    else
        y = IntegralLimit_f * multiplier;
    end
end

== matlab function gtcs_model_and_controller/CONTROLLER/CURRENT PID/Output Deadband Compensator ==
  data: u input; y output; OutputDeadband_f input
function y = Output_Deadband_Compensator(u, OutputDeadband_f)
    if u==0
        multiplier = 1;
    else
        multiplier = floor(u/abs(u));
    end
    if abs(u) == 0
        y = 0;
    else
        y = u + OutputDeadband_f * multiplier;
    end
end

== matlab function gtcs_model_and_controller/BLDC MOTOR + GEARBOX + LOAD/Drive Logic ==
  data: theta input; AH output; AL output; BH output; BL output; CH output; CL output
function [AH,AL,BH,BL,CH,CL] = fun_driveLogic(theta)
    AH = 0;AL = 0;BH = 0;BL = 0;CH = 0;CL = 0;
    if theta>=0 && theta<60
        AH = 1;
        BL = 1;
    elseif theta>=60 && theta<120
        AH = 1;
        CL = 1;
    elseif theta>=120 && theta<180
        BH = 1;
        CL = 0;
    elseif theta>=180 && theta<240
        AL = 1;
        BH = 1;
    elseif theta>=240 && theta<300
        AL = 1;
        CH = 1;
    elseif theta>=300 && theta<=360
        BL = 1;
        CH = 1;
    end
end
